simulink model "Process_PLC"  (R2022b)
settings: Solver=VariableStepAuto  StartTime=0.0  StopTime=10.0  RelTol=1e-3
undefined symbols (not defined in the file): A, Q
settings Model: Creator=karnbongkotboonriong  LastModifiedBy=karnbongkotboonriong

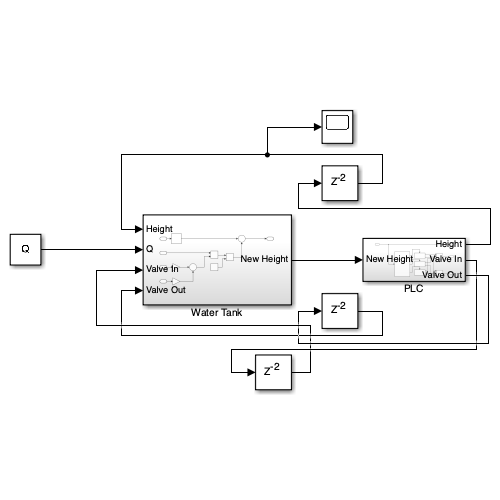
[thumbnail: Simulink's stored preview of the top-level diagram]
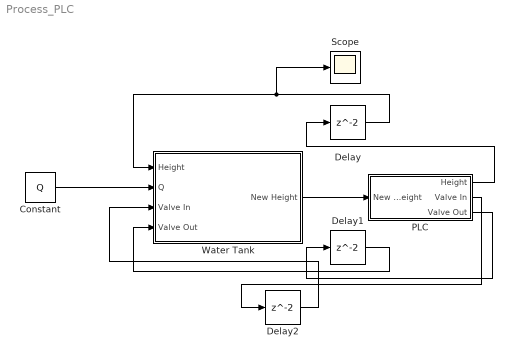
== system Process_PLC ==
  Constant : Constant  Value=Q
  Delay : Delay
  Delay1 : Delay
  Delay2 : Delay
  PLC : Subsystem
  Scope : Scope
  Water Tank : Subsystem
  wires:
  Delay/1 -> Scope/1, Water Tank/1(Height)
  Delay2/1 -> Water Tank/3(Valve In)
  Constant/1 -> Water Tank/2(Q)
  Delay1/1 -> Water Tank/4(Valve Out)
  PLC/2(Valve In) -> Delay2/1
  Water Tank/1(New Height) -> PLC/1(New Height)
  PLC/3(Valve Out) -> Delay1/1
  PLC/1(Height) -> Delay/1

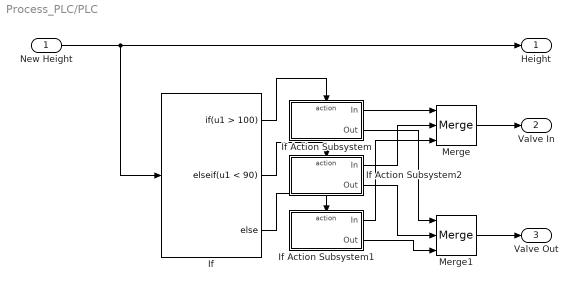
== system Process_PLC/PLC ==
  New Height : Inport
  If : If  IfExpression=u1 > 100  ElseIfExpressions=u1 < 90
  If Action Subsystem : Subsystem  TreatAsAtomicUnit=on
  If Action Subsystem1 : Subsystem  TreatAsAtomicUnit=on
  If Action Subsystem2 : Subsystem  TreatAsAtomicUnit=on
  Merge : Merge  Inputs=3
  Merge1 : Merge  Inputs=3
  Height : Outport
  Valve In : Outport  Port=2
  Valve Out : Outport  Port=3
  wires:
  New Height/1 -> If/1, Height/1
  Merge1/1 -> Valve Out/1
  Merge/1 -> Valve In/1
  If/2 -> If Action Subsystem2/Action
  If/3 -> If Action Subsystem1/Action
  If Action Subsystem/1(In) -> Merge/1
  If Action Subsystem2/1(In) -> Merge/2
  If Action Subsystem1/1(In) -> Merge/3
  If Action Subsystem/2(Out) -> Merge1/1
  If Action Subsystem2/2(Out) -> Merge1/2
  If Action Subsystem1/2(Out) -> Merge1/3
  If/1 -> If Action Subsystem/Action

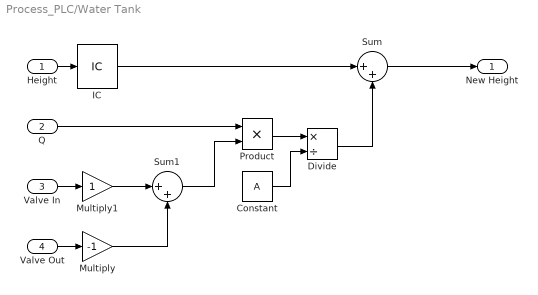
== system Process_PLC/Water Tank ==
  Height : Inport
  Q : Inport  Port=2
  Valve In : Inport  Port=3
  Valve Out : Inport  Port=4
  Constant : Constant  Value=A
  Divide : Product  Inputs=*/
  IC : InitialCondition  Value=0
  Multiply : Gain  Gain=-1
  Multiply1 : Gain
  Product : Product
  Sum : Sum  Inputs=|++
  Sum1 : Sum  Inputs=|++
  New Height : Outport
  wires:
  Valve Out/1 -> Multiply/1
  Valve In/1 -> Multiply1/1
  Multiply/1 -> Sum1/2
  Multiply1/1 -> Sum1/1
  Sum1/1 -> Product/2
  Q/1 -> Product/1
  Product/1 -> Divide/1
  Constant/1 -> Divide/2
  Divide/1 -> Sum/2
  Sum/1 -> New Height/1
  Height/1 -> IC/1
  IC/1 -> Sum/1

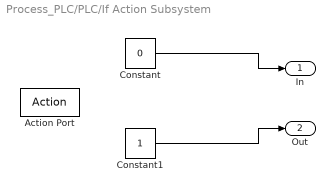
== system Process_PLC/PLC/If Action Subsystem ==
  Action Port : ActionPort
  Constant : Constant  Value=0
  Constant1 : Constant
  In : Outport
  Out : Outport  Port=2
  wires:
  Constant/1 -> In/1
  Constant1/1 -> Out/1

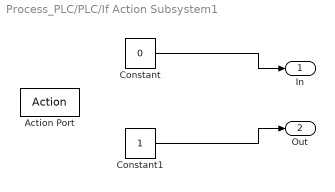
== system Process_PLC/PLC/If Action Subsystem1 ==
  Action Port : ActionPort
  Constant : Constant  Value=0
  Constant1 : Constant
  In : Outport
  Out : Outport  Port=2
  wires:
  Constant/1 -> In/1
  Constant1/1 -> Out/1

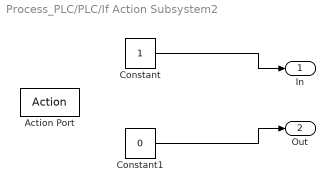
== system Process_PLC/PLC/If Action Subsystem2 ==
  Action Port : ActionPort
  Constant : Constant
  Constant1 : Constant  Value=0
  In : Outport
  Out : Outport  Port=2
  wires:
  Constant/1 -> In/1
  Constant1/1 -> Out/1
